simulink model "sgMdl_MQTT_Loopback"  (R2024b)
settings: Solver=FixedStepAuto  StartTime=0.0  StopTime=inf  RelTol=1e-3  EnableMultiTasking=on
libraries: speedgoatlib_mqtt x6, simulink x3
Description:
  | MQTT Loopback
settings Model: sg_rtwmakecfg_data=_sg_IO75X_v1_2_0__sg_netxLib_MSVC140_  ModifiedByFormat=Speedgoat  Creator=Speedgoat  LastModifiedBy=Speedgoat
settings SolverCC: ConcurrentTasks=on  AlgebraicLoopSolver=TrustRegion  PositivePriorityOrder=on  AutoInsertRateTranBlk=on  InsertRTBMode=Never (minimum delay)  MaxZcPerStep=1
settings DataIOCC: LimitDataPoints=on  SaveFormat=StructureWithTime  ReturnWorkspaceOutputs=off
settings OptimizationCC: BlockReduction=off  BooleanDataType=off  OptimizeBlockIOStorage=off  BufferReuse=off  ReuseModelBlockBuffer=off  GlobalBufferReuse=off  ExpressionFolding=off  LocalBlockOutputs=off  OptimizeDataStoreBuffers=off  BusAssignmentInplaceUpdate=off
settings DebuggingCC: SaveWithParameterizedLinksMsg=none  UnderspecifiedInitializationDetection=Classic  MergeDetectMultiDrivingBlocksExec=none  SignalResolutionControl=TryResolveAllWithWarning  TasksWithSamePriorityMsg=none  ParameterOverflowMsg=warning  UnconnectedInputMsg=warning  UnconnectedOutputMsg=warning  UnconnectedLineMsg=warning  SFUnexpectedBacktrackingDiag=warning  SFNoUnconditionalDefaultTransitionDiag=warning  SFExecutionAtInitializationDiag=none  ArithmeticOperatorsInVariantConditions=warning
settings HardwareCC: ProdBitPerLong=64  ProdLongLongMode=on  ProdHWDeviceType=Intel->x86-64 (Linux 64)  TargetBitPerPointer=64  TargetBitPerSizeT=64  TargetBitPerPtrDiffT=64  TargetLongLongMode=on  TargetIntDivRoundTo=Zero  TargetEndianess=LittleEndian  TargetWordSize=64  TargetHWDeviceType=MATLAB Host
settings ModelReferenceCC: EnableRefExpFcnMdlSchedulingChecks=on  PropagateSignalLabelsOutOfModel=off
settings SFSimCC: SimUseLocalCustomCode=off  CustomCodeUndefinedFunction=UseInterfaceOnly
settings RTWCC: Description=Speedgoat Real-Time Target Machine  SystemTargetFile=speedgoat.tlc  TemplateMakefile=slrealtime_default_tmf  RetainRTWFile=on  RTWUseLocalCustomCode=off  Toolchain=Simulink Real-Time Toolchain  BuildConfiguration=Faster Runs  TargetLang=C++  GPUComputeCapability=3.5  DLArmComputeVersion=19.05
settings CodeAppCC: StateflowObjectComments=on
settings SimulinkRealTimeTargetCC: SubcomponentCodeInterfacePackaging=Reusable function  InstructionSetFMA=off  LogToMDFFile=off  SLRTFileLogMaxRuns=10  UseGCCFastMath=on
settings ConfigComp: CovMetricSettings=dw  CovSaveCumulativeToWorkspaceVar=on  CovSaveSingleToWorkspaceVar=on  CovExternalEMLEnable=off  CovBoundaryAbsTol=1.0e-5

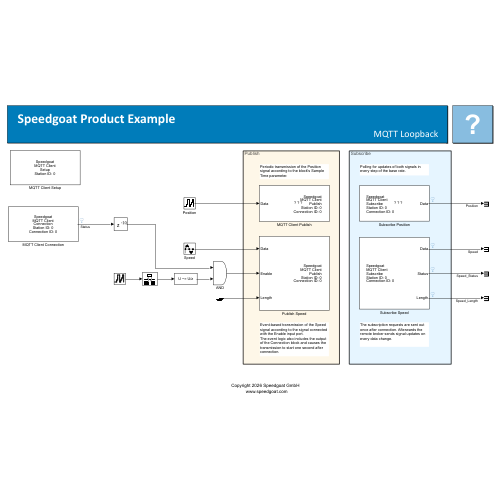
[thumbnail: Simulink's stored preview of the top-level diagram]
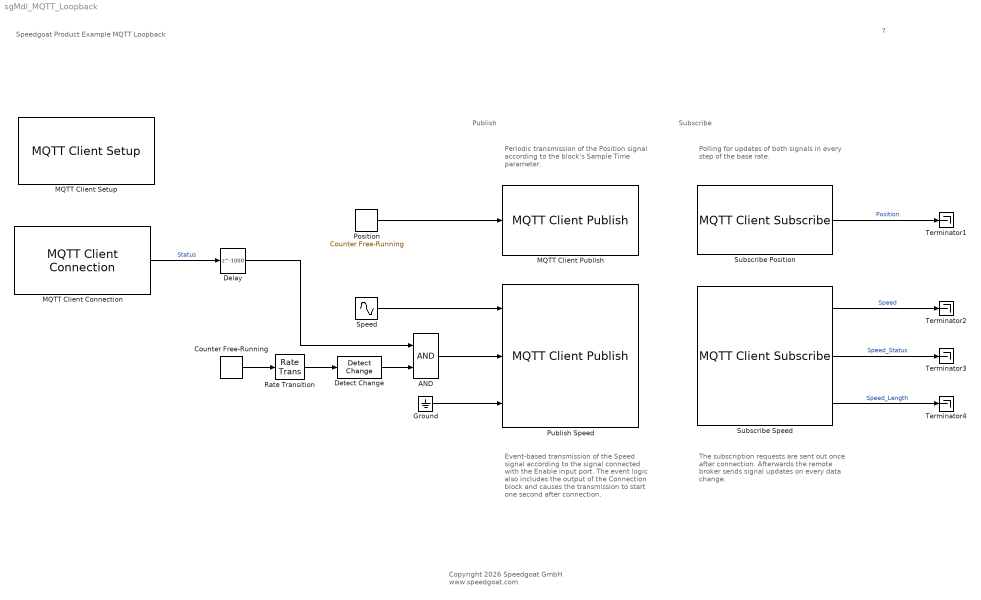
== system sgMdl_MQTT_Loopback ==
  note: Subscribe
  note: Periodic transmission of the Position signal according to the block's Sample Time parameter.
  note: Publish
  note: Event-based transmission of the Speed signal according to the signal connected with the Enable input port.
      | The event logic also includes the output of the Connection block and causes the transmission to start one second after connection.
  note: Polling for updates of both signals in every step of the base rate.
  note: The subscription requests are sent out once after connection. Afterwards the remote broker sends signal updates on every data change.
  note: Speedgoat Product Example
      | MQTT Loopback
  note: ?
  note: Copyright 2026 Speedgoat GmbH
      |  www.speedgoat.com
  AND : Logic  IconShape=distinctive  AllPortsSameDT=off  OutDataTypeStr=boolean
  Counter Free-Running : simulink/Sources/Counter Free-Running  NumBits=16  tsamp=1
  Delay : Delay  DelayLength=1000
  Detect Change : simulink/Logic and Bit Operations/Detect Change  vinit=0  OutDataTypeStr=boolean
  Ground : Ground
  MQTT Client Connection : speedgoatlib_mqtt/Client/MQTT Client Connection  StationId=0  ConnectionId=0  IpAddrStr='192.168.10.50'  TcpPort=1883  SampleTime=0.001  UserAuthentication=off  Username=''  Password=''
      settings: SourceProductName=Simulink Real-Time: Speedgoat I/O Blockset
  MQTT Client Publish : speedgoatlib_mqtt/Client/MQTT Client Publish  ClientId=0  ConnectionId=0  Topic='position'  QoS=2 - exactly once  Retain=on  Extended=off  SampleTime=1
      settings: SourceProductName=Simulink Real-Time: Speedgoat I/O Blockset
  MQTT Client Setup : speedgoatlib_mqtt/Client/MQTT Client Setup  StationId=0  ClientIdentifier='client1'  IpAddrStr='192.168.10.1'
      settings: SourceProductName=Simulink Real-Time: Speedgoat I/O Blockset
  Position : simulink/Sources/Counter Free-Running  NumBits=32  tsamp=-1
  Publish Speed : speedgoatlib_mqtt/Client/MQTT Client Publish  ClientId=0  ConnectionId=0  Topic='speed'  QoS=0 - at most once  Retain=off  Extended=on  SampleTime=0.001
      settings: SourceProductName=Simulink Real-Time: Speedgoat I/O Blockset
  Rate Transition : RateTransition
  Speed : Sin  SineType=Sample based  Amplitude=100  Frequency=2*pi  Phase=pi  Samples=10000  SampleTime=0.001
  Subscribe Position : speedgoatlib_mqtt/Client/MQTT Client Subscribe  ClientId=0  ConnectionId=0  Topic='position'  QoS=2 - exactly once  InitValue=uint32(0)  Extended=off  SampleTime=0.001
      settings: SourceProductName=Simulink Real-Time: Speedgoat I/O Blockset
  Subscribe Speed : speedgoatlib_mqtt/Client/MQTT Client Subscribe  ClientId=0  ConnectionId=0  Topic='speed'  QoS=0 - at most once  InitValue=0  Extended=on  SampleTime=0.001
      settings: SourceProductName=Simulink Real-Time: Speedgoat I/O Blockset
  Terminator{1..4} (4 alike) : Terminator
  wires:
  MQTT Client Connection/1 -> Delay/1  "Status"
  Subscribe Position/1 -> Terminator1/1  "Position"
  Counter Free-Running/1 -> Rate Transition/1
  Subscribe Speed/1 -> Terminator2/1  "Speed"
  Subscribe Speed/2 -> Terminator3/1  "Speed_Status"
  Subscribe Speed/3 -> Terminator4/1  "Speed_Length"
  Rate Transition/1 -> Detect Change/1
  Speed/1 -> Publish Speed/1
  AND/1 -> Publish Speed/2
  Detect Change/1 -> AND/2
  Position/1 -> MQTT Client Publish/1
  Delay/1 -> AND/1
  Ground/1 -> Publish Speed/3
